simulink model "PamSIMULAB02"  (R2016a)
settings: Solver=VariableStepAuto  StartTime=0.0  StopTime=10.0  RelTol=1e-3
libraries: dsparch4 x1, dspsigops x1
settings Model: Creator=ahpar  LastModifiedBy=ahpar

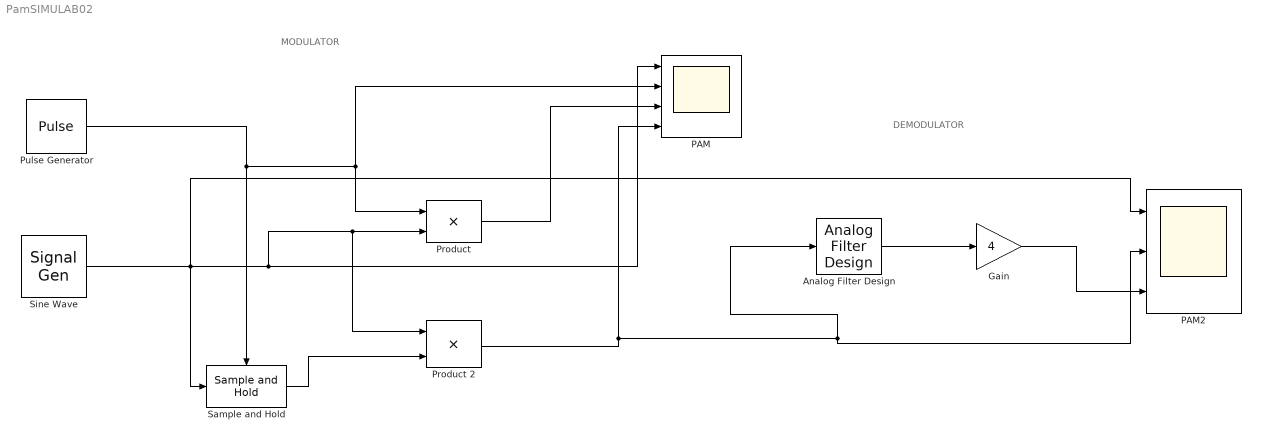
== system PamSIMULAB02 ==
  note: MODULATOR
  note: DEMODULATOR
  Analog Filter Design : dsparch4/Analog Filter Design  method=Chebyshev I  filttype=Lowpass  N=8  Wlo=(2*pi)*2.5  Whi=80  Rp=2  Rs=40
  Gain : Gain  Gain=4
  PAM : Scope  NumInputPorts=4
  PAM2 : Scope  NumInputPorts=3
  Product : Product
  Product 2 : Product
  Pulse Generator : DiscretePulseGenerator  PulseType=Time based  Period=0.2  PulseWidth=25
  Sample and Hold : dspsigops/Sample and Hold  trig=Rising edge  initCond=0  latchinput=off
  Sine Wave : SignalGenerator  Amplitude=0.9  Frequency=2  Units=rad/sec
  wires:
  Sine Wave/1 -> PAM2/1, Sample and Hold/1, Product 2/1, Product/2, PAM/1
  Pulse Generator/1 -> Sample and Hold/Trigger, PAM/2, Product/1
  Product/1 -> PAM/3
  Sample and Hold/1 -> Product 2/2
  Product 2/1 -> Analog Filter Design/1, PAM2/2, PAM/4
  Gain/1 -> PAM2/3
  Analog Filter Design/1 -> Gain/1
